simulink model "Fig318"  (R2014b)
settings: Solver=ode3  StartTime=0.0  StopTime=10.007  FixedStep=2e-6  RelTol=1e-5
libraries: commfilt2 x4, commutil2 x2, commchan3 x1, commsink2 x1, commanapbnd3 x1, commrandsrc2 x1
settings Model: Creator=Dennis Silage  LastModifiedBy=Silage
settings DataIOCC: SignalLoggingSaveFormat=ModelDataLogs
settings OptimizationCC: ExpressionDepthLimit=2147483647  InitFltsAndDblsToZero=on  EfficientMapNaN2IntZero=off
settings DebuggingCC: UnderspecifiedInitializationDetection=Classic  MergeDetectMultiDrivingBlocksExec=none  SolverPrmCheckMsg=none  FcnCallInpInsideContextMsg=UseLocalSettings  StateNameClashWarn=warning
settings HardwareCC: TargetIntDivRoundTo=Zero  TargetEndianess=LittleEndian  TargetHWDeviceType=MATLAB Host  ProdEqTarget=off
settings CodeAppCC: MaxIdLength=128
settings GRTTargetCC: CombineOutputUpdateFcns=off  GRTInterface=on

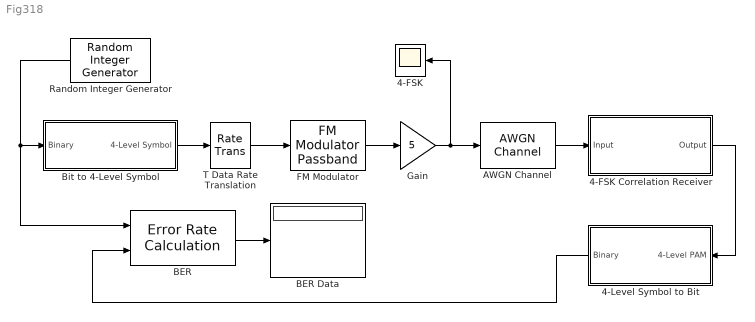
== system Fig318 ==
  4-FSK : Scope
      settings: TimeRange=0.008  YMin=-6  YMax=6
  4-FSK Correlation Receiver : Subsystem
  4-Level Symbol to Bit : Subsystem
  AWGN Channel : commchan3/AWGN Channel  InputProcessing=Inherited (this choice will be removed - see release notes)  seed=randseed  noiseMode="Signal to noise ratio  (Eb/No)"  EbNodB=50  EsNodB=20  SNRdB=10  bitsPerSym=2  Ps=12.5  Tsym=2e-3  variance=0
  BER : commsink2/Error Rate Calculation  N=8  st_delay=0  cp_mode=Entire frame  subframe=[]  PMode=Port  WsName=ErrorVec  RsMode2=off  stop=off  numErr=100  maxBits=1e6
  BER Data : Display
  Bit to 4-Level Symbol : Subsystem
  FM Modulator : commanapbnd3/FM Modulator Passband  Fc=20000  Ph=-pi/2  Kc=1000
  Gain : Gain  Gain=5
  Random Integer Generator : commrandsrc2/Random Integer Generator  mul=2  seed=46  Ts=1e-3  frameBased=off  sampPerFrame=1  orient=off  outDataType=double
  T Data Rate Translation : RateTransition  OutPortSampleTime=2e-6
  wires:
  BER/1 -> BER Data/1
  AWGN Channel/1 -> 4-FSK Correlation Receiver/1(Input)
  T Data Rate Translation/1 -> FM Modulator/1
  Bit to 4-Level Symbol/1(4-Level Symbol) -> T Data Rate Translation/1
  FM Modulator/1 -> Gain/1
  Gain/1 -> AWGN Channel/1, 4-FSK/1
  Random Integer Generator/1 -> Bit to 4-Level Symbol/1(Binary), BER/1
  4-FSK Correlation Receiver/1(Output) -> 4-Level Symbol to Bit/1(4-Level PAM)
  4-Level Symbol to Bit/1(Binary) -> BER/2

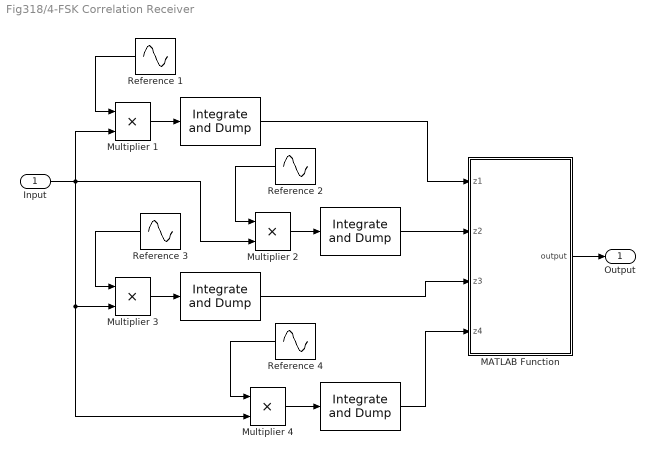
== system Fig318/4-FSK Correlation Receiver ==
  Input : Inport
  " " : commfilt2/Integrate and Dump  obssamples=1000  offsetsamples=0  nodump=off  roundingMode=Floor  overflowMode=off
  "  " : commfilt2/Integrate and Dump  obssamples=1000  offsetsamples=0  nodump=off  roundingMode=Floor  overflowMode=off
  "   " : commfilt2/Integrate and Dump  obssamples=1000  offsetsamples=0  nodump=off  roundingMode=Floor  overflowMode=off
  "      " : commfilt2/Integrate and Dump  obssamples=1000  offsetsamples=0  nodump=off  roundingMode=Floor  overflowMode=off
  MATLAB Function : MATLAB Function  TreatAsAtomicUnit=on
  Multiplier {1..4} (4 alike) : Product  RndMeth=Zero
  Reference 1 : Sin  Amplitude=5  Frequency=46000*pi  SampleTime=2e-6
  Reference 2 : Sin  Amplitude=5  Frequency=42000*pi  SampleTime=2e-6
  Reference 3 : Sin  Amplitude=5  Frequency=38000*pi  SampleTime=2e-6
  Reference 4 : Sin  Amplitude=5  Frequency=34000*pi  SampleTime=2e-6
  Output : Outport
  wires:
  Multiplier 1/1 -> " "/1
  Reference 1/1 -> Multiplier 1/1
  Multiplier 2/1 -> "  "/1
  Reference 2/1 -> Multiplier 2/1
  Multiplier 3/1 -> "   "/1
  Reference 3/1 -> Multiplier 3/1
  Multiplier 4/1 -> "      "/1
  Input/1 -> Multiplier 1/2, Multiplier 2/2, Multiplier 3/2, Multiplier 4/2
  Reference 4/1 -> Multiplier 4/1
  " "/1 -> MATLAB Function/1(z1)
  "  "/1 -> MATLAB Function/2(z2)
  "   "/1 -> MATLAB Function/3(z3)
  "      "/1 -> MATLAB Function/4(z4)
  MATLAB Function/1(output) -> Output/1

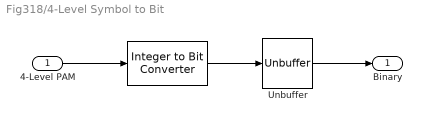
== system Fig318/4-Level Symbol to Bit ==
  4-Level PAM : Inport
  " " : commutil2/Integer to Bit Converter  nbits=2  signedInputValues=Unsigned  bitOrder=MSB first  outDtype=Inherit via internal rule
  Unbuffer : Unbuffer  SampleBasedProcessing=Same as frame based
  Binary : Outport
  wires:
  " "/1 -> Unbuffer/1
  Unbuffer/1 -> Binary/1
  4-Level PAM/1 -> " "/1

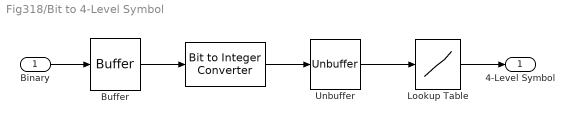
== system Fig318/Bit to 4-Level Symbol ==
  Binary : Inport
  " " : commutil2/Bit to Integer Converter  nbits=2  bitOrder=MSB first  signedOutputValues=Unsigned  outDtype=Inherit via internal rule  outDtypeSigned=Inherit via internal rule
  Buffer : Buffer  N=2  TreatMby1Signals=One channel
  Lookup Table : Lookup_n-D  NumberOfTableDimensions=1  BreakpointsForDimension1=[0, 1, 2, 3]  BreakpointsForDimension3=[5, 7]  BreakpointsForDimension1DataTypeStr=double  IndexSearchMethod=Linear search  Table=[-3, -1, 1, 3]  TableDataTypeStr=double  InternalRulePriority=Speed  OutDataTypeStr=double  RndMeth=Simplest  InputSameDT=on
  Unbuffer : Unbuffer  SampleBasedProcessing=Same as frame based
  4-Level Symbol : Outport
  wires:
  Lookup Table/1 -> 4-Level Symbol/1
  Binary/1 -> Buffer/1
  Buffer/1 -> " "/1
  " "/1 -> Unbuffer/1
  Unbuffer/1 -> Lookup Table/1

== matlab function Fig318/4-FSK Correlation Receiver/MATLAB Function ==
  data: z1 input; output output; z2 input; z3 input; z4 input
function output = fcn(z1, z2, z3, z4)
%#codegen
output = -1;
if (z1 > z2) && (z1 > z3) && (z1 > z4)
    output = 3;     %z1 is greatest
end
if output < 0
    if (z2 > z1) && (z2 > z3) && (z2 > z4)
        output = 2; %z2 is greatest
    end
end
if output < 0
    if (z3 > z1) && (z3 > z2) && (z3 > z4)
        output = 1; %z3 is greatest
    end
end
if output < 0
    output = 0;     %z4 is greatest 
end
